simulink model "Gear_lab3"  (R2024b)
settings: Solver=VariableStepAuto  StartTime=0.0  StopTime=Sim_Time  RelTol=1e-3
undefined symbols (not defined in the file): b, J, k
settings Model: Creator=ACER NITRO 5  LastModifiedBy=ACER NITRO 5

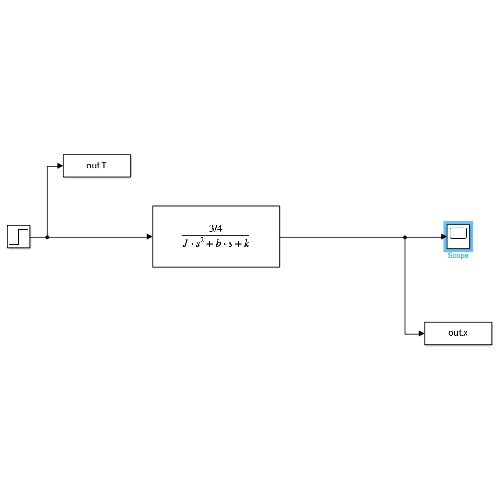
[thumbnail: Simulink's stored preview of the top-level diagram]
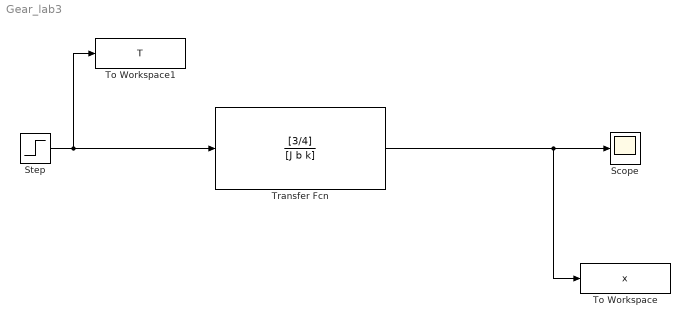
== system Gear_lab3 ==
  Scope : Scope
  Step : Step  SampleTime=0
  To Workspace : ToWorkspace  VariableName=x  SaveFormat=Timeseries  SampleTime=-1
  To Workspace1 : ToWorkspace  VariableName=T  SaveFormat=Timeseries  SampleTime=-1
  Transfer Fcn : TransferFcn  Numerator=[3/4]  Denominator=[J b k]
  wires:
  Step/1 -> To Workspace1/1, Transfer Fcn/1
  Transfer Fcn/1 -> Scope/1, To Workspace/1
